simulink library "tpm"  (R2021b)
settings: Solver=VariableStepAuto  StartTime=0.0  StopTime=10.0  RelTol=1e-3
undefined symbols (not defined in the file or in its folder): ENUM_AN_LF, ENUM_AN_LR, ENUM_AN_RF, ENUM_AN_RR, ENUM_POWERSTA_OFF, ENUM_POWERSTA_OFFA, ENUM_POWERSTA_OFFC, ENUM_POWERSTA_ON, ENUM_POWERSTA_READY, ENUM_POWERSTA_STANDBY, ENUM_PWRSTASW_OFF, ENUM_PWRSTASW_OFFA, ENUM_PWRSTASW_OFFCHVCHRG, ENUM_PWRSTASW_STANDBY, FALSE, KTPM_Delay_raw8, KTPM_WhlRotDir_enum_ovrdflg, KTPM_WhlRotDir_enum_ovrdval, TRUE, ZERO_FLOAT, ZERO_INT
libraries: simulink x58, hcu_lib x25, $bdroot x18
(part 8 of 8)

== stateflow chart tpm/TPM/TPMS/TPMS/Learn/AutoLocation/Doublecheck/Chart ==
  (default) -> (junction 18)
  (junction 18) -> (junction 19) [order 1] : [VTPM_SaveToRAM_flg]
  (junction 18) -> (junction 36) [order 2]
  (junction 19) -> (junction 23) : {
      |  VTPM_ChkLFID_raw=VTPM_LFID_raw;
      |  VTPM_ChkRFID_raw=VTPM_RFID_raw;
      |  VTPM_ChkLRID_raw=VTPM_LRID_raw;
      |  VTPM_ChkRRID_raw=VTPM_RRID_raw;
      | }
  (junction 23) -> (junction 36)
  data: VTPM_LFID_raw input; VTPM_RFID_raw input; VTPM_LRID_raw input; VTPM_RRID_raw input; VTPM_ChkLFID_raw output uint32; VTPM_ChkRFID_raw output uint32; VTPM_ChkLRID_raw output uint32; VTPM_ChkRRID_raw output uint32; VTPM_SaveToRAM_flg input

== stateflow chart tpm/TPM/TPMS/TPMS/Learn/AutoLocation/IDIdentify/Subsystem1/Chart1 ==
  state GCal [parallel]
    settings: executionOrder=1
    state NoSignal
      en:G=false;
    state SignalIn
      en:G=true;
    (default) -> NoSignal
    NoSignal -> (junction 17) : [VINP_DATAin_flg]
    (junction 17) -> SignalIn [order 1] : [!Used]
    (junction 17) -> (junction 19) [order 2]
    (junction 19) -> NoSignal [order 2]
    (junction 19) -> SignalIn [order 1] : [VINP_IDin_raw32==IDout]
    SignalIn -> NoSignal
  state IDCheck [parallel]
    settings: executionOrder=2
    state Unused
      en:IDout=0;
      VTPM_S2IDLock_flg=false;
      Used=false;
      IDLock_cnt=0;
    state FlashID
      en:
      IDout=VINP_S2ID_raw;
      Used=true;
      VTPM_S2IDLock_flg=true;
    state VINP_DATAin_flg
      state Used
        en:IDout=VINP_IDin_raw32;
        Used=true;
        IDLock_cnt+=1;
      state Lock
        en:VTPM_S2IDLock_flg=true;
      Used -> Used [order 2] : [VINP_DATAin_flg&&IDout==VINP_IDin_raw32]
      Used -> Lock [order 1] : [IDLock_cnt>=4]
    (default) -> Unused
    Unused -> FlashID [order 1] : [VTPM_FlashIDlock_flg]
    FlashID -> Unused : [VINP_TPMSResButt_flg]
    Unused -> Used [order 2] : [VINP_DATAin_flg]
    Used -> Unused [order 3] : [VTPM_S2timeout_flg==1]
    VINP_DATAin_flg -> Unused : [VINP_TPMSResButt_flg]
  state timecounter [parallel]
    settings: executionOrder=3
    state standby
      en:
      VTPM_S2timeout_flg=0;
      VTPM_timeout_cnt=0;
    state counter
      during:
      VTPM_timeout_cnt=VTPM_timeout_cnt+1;
    state stopcounter
    state timeout
      en:
      VTPM_S2timeout_flg=1;
    (default) -> standby
    (junction 76) -> standby
    (junction 74) -> (junction 76)
    standby -> counter : [Used&&!VTPM_FlashIDlock_flg]
    counter -> standby [order 1] : [!Used||(VINP_DATAin_flg&&IDout==VINP_IDin_raw32)]
    stopcounter -> counter : [VINP_VehSpeed_kph>=20]
    counter -> stopcounter [order 3] : [VINP_VehSpeed_kph<20]
    counter -> timeout [order 2] : [VTPM_timeout_cnt>12000]
    timeout -> (junction 74)
  data: VINP_IDin_raw32 input; VINP_TPMSResButt_flg input; VINP_DATAin_flg input; G output boolean; Used output boolean; VTPM_S2IDLock_flg output boolean; IDout output uint32; VTPM_FlashIDlock_flg input; VINP_S2ID_raw input; VINP_VehSpeed_kph input; IDLock_cnt local uint32; VTPM_timeout_cnt local uint32; VTPM_S2timeout_flg output boolean

== matlab function tpm/TPM/TPMS/TPMS/Learn/AutoLocation/IDIdentify/Subsystem1/Enabled Subsystem1/MATLAB Function ==
  data: C input; S output; Min input; X2 input; X3 input; X4 input; Y2 output; Y3 output; Y4 output; X5 input; X6 input; X7 input; X8 input; X9 input; Y5 output; Y6 output; Y7 output; Y8 output; Y9 output
function [S,Y2,Y3,Y4,Y5,Y6,Y7,Y8,Y9]   = fcn(C,Min,X2,X3,X4,X5,X6,X7,X8,X9)
Y=int16([X2 X3 X4 X5 X6 X7 X8 X9 Min]);
if (C<9)
    S=300;
else
    B=sort(Y);
    D=zeros(1,length(B));
    for i=1:1:length(D)
        if (i~=length(D))
            D(i)=B(i+1)-B(i);
        else
            if (B(length(D))-B(1)>B(1)+96-B(length(D)))
                D(length(D))=B(1)+96-B(length(D));
            else
                D(length(D))=B(length(D))-B(1);
            end
        end
    end

    [K,I]=sort(D);
    S=sum(K(1:7));
end
Y2=Y(2);
Y3=Y(3);
Y4=Y(4);
Y5=Y(5);
Y6=Y(6);
Y7=Y(7);
Y8=Y(8);
Y9=Y(9);

== matlab function tpm/TPM/TPMS/TPMS/Learn/AutoLocation/IDIdentify/Subsystem1/Enabled Subsystem2/MATLAB Function ==
  data: C input; S output; Min input; X2 input; X3 input; X4 input; Y2 output; Y3 output; Y4 output; X5 input; X6 input; X7 input; X8 input; X9 input; Y5 output; Y6 output; Y7 output; Y8 output; Y9 output
function [S,Y2,Y3,Y4,Y5,Y6,Y7,Y8,Y9]   = fcn(C,Min,X2,X3,X4,X5,X6,X7,X8,X9)
Y=int16([X2 X3 X4 X5 X6 X7 X8 X9 Min]);
if (C<9)
    S=300;
else
    B=sort(Y);
    D=zeros(1,length(B));
    for i=1:1:length(D)
        if (i~=length(D))
            D(i)=B(i+1)-B(i);
        else
            if (B(length(D))-B(1)>B(1)+96-B(length(D)))
                D(length(D))=B(1)+96-B(length(D));
            else
                D(length(D))=B(length(D))-B(1);
            end
        end
    end

    [K,I]=sort(D);
    S=sum(K(1:7));
end
Y2=Y(2);
Y3=Y(3);
Y4=Y(4);
Y5=Y(5);
Y6=Y(6);
Y7=Y(7);
Y8=Y(8);
Y9=Y(9);

== matlab function tpm/TPM/TPMS/TPMS/Learn/AutoLocation/IDIdentify/Subsystem1/Enabled Subsystem3/MATLAB Function ==
  data: C input; S output; Min input; X2 input; X3 input; X4 input; Y2 output; Y3 output; Y4 output; X5 input; X6 input; X7 input; X8 input; X9 input; Y5 output; Y6 output; Y7 output; Y8 output; Y9 output
function [S,Y2,Y3,Y4,Y5,Y6,Y7,Y8,Y9]   = fcn(C,Min,X2,X3,X4,X5,X6,X7,X8,X9)
Y=int16([X2 X3 X4 X5 X6 X7 X8 X9 Min]);
if (C<9)
    S=300;
else
    B=sort(Y);
    D=zeros(1,length(B));
    for i=1:1:length(D)
        if (i~=length(D))
            D(i)=B(i+1)-B(i);
        else
            if (B(length(D))-B(1)>B(1)+96-B(length(D)))
                D(length(D))=B(1)+96-B(length(D));
            else
                D(length(D))=B(length(D))-B(1);
            end
        end
    end

    [K,I]=sort(D);
    S=sum(K(1:7));
end
Y2=Y(2);
Y3=Y(3);
Y4=Y(4);
Y5=Y(5);
Y6=Y(6);
Y7=Y(7);
Y8=Y(8);
Y9=Y(9);

== matlab function tpm/TPM/TPMS/TPMS/Learn/AutoLocation/IDIdentify/Subsystem1/Enabled Subsystem5/MATLAB Function ==
  data: C input; S output; Min input; X2 input; X3 input; X4 input; Y2 output; Y3 output; Y4 output; X5 input; X6 input; X7 input; X8 input; X9 input; Y5 output; Y6 output; Y7 output; Y8 output; Y9 output
function [S,Y2,Y3,Y4,Y5,Y6,Y7,Y8,Y9]   = fcn(C,Min,X2,X3,X4,X5,X6,X7,X8,X9)
Y=int16([X2 X3 X4 X5 X6 X7 X8 X9 Min]);
if (C<9)
    S=300;
else
    B=sort(Y);
    D=zeros(1,length(B));
    for i=1:1:length(D)
        if (i~=length(D))
            D(i)=B(i+1)-B(i);
        else
            if (B(length(D))-B(1)>B(1)+96-B(length(D)))
                D(length(D))=B(1)+96-B(length(D));
            else
                D(length(D))=B(length(D))-B(1);
            end
        end
    end

    [K,I]=sort(D);
    S=sum(K(1:7));
end
Y2=Y(2);
Y3=Y(3);
Y4=Y(4);
Y5=Y(5);
Y6=Y(6);
Y7=Y(7);
Y8=Y(8);
Y9=Y(9);

== stateflow chart tpm/TPM/TPMS/TPMS/Send/DATA/Chart ==
  state read
    (default) -> (junction 7) : {
        | VTPM_PreS1Pressure_raw=VINP_FlashLFWheelPress_raw8;
        | VTPM_PreS2Pressure_raw=VINP_FlashRFWheelPress_raw8;
        | VTPM_PreS3Pressure_raw=VINP_FlashLRWheelPress_raw8;
        | VTPM_PreS4Pressure_raw=VINP_FlashRRWheelPress_raw8;
        | VTPM_PreS1Temp_raw=VINP_FlashLFWheelTemp_C;
        | VTPM_PreS2Temp_raw=VINP_FlashRFWheelTemp_C;
        | VTPM_PreS3Temp_raw=VINP_FlashLRWheelTemp_C;
        | VTPM_PreS4Temp_raw=VINP_FlashRRWheelTemp_C;
        | }
    read -> (junction 7) : [VINP_DATAin_flg||VINP_TPMSResButt_flg]
    (junction 7) -> (junction 9) [order 1] : [VINP_IDin_raw32==VTPM_S1ID_raw32&&VTPM_IDLOCK_flg&&VINP_DATAin_flg]
    (junction 7) -> (junction 11) [order 2]
    (junction 9) -> (junction 27) : {VTPM_PreS1Pressure_raw=VINP_Pin_raw8;
        |  VTPM_PreS1Temp_raw=VINP_Tin_raw8;
        |  VTPM_PreS1readdone_flg=true;
        | }
    (junction 11) -> (junction 13) [order 1] : [VINP_IDin_raw32==VTPM_S2ID_raw32&&VTPM_IDLOCK_flg&&VINP_DATAin_flg]
    (junction 11) -> (junction 15) [order 2]
    (junction 13) -> (junction 30) : {VTPM_PreS2Pressure_raw=VINP_Pin_raw8;
        |  VTPM_PreS2Temp_raw=VINP_Tin_raw8;
        |  VTPM_PreS2readdone_flg=true;
        | }
    (junction 15) -> (junction 17) [order 1] : [VINP_IDin_raw32==VTPM_S3ID_raw32&&VTPM_IDLOCK_flg&&VINP_DATAin_flg]
    (junction 15) -> (junction 19) [order 2]
    (junction 17) -> (junction 32) : {VTPM_PreS3Pressure_raw=VINP_Pin_raw8;
        |  VTPM_PreS3Temp_raw=VINP_Tin_raw8;
        |  VTPM_PreS3readdone_flg=true;
        | }
    (junction 19) -> (junction 21) [order 1] : [VINP_IDin_raw32==VTPM_S4ID_raw32&&VTPM_IDLOCK_flg&&VINP_DATAin_flg]
    (junction 19) -> (junction 25) [order 2]
    (junction 21) -> (junction 34) : {VTPM_PreS4Pressure_raw=VINP_Pin_raw8;
        |  VTPM_PreS4Temp_raw=VINP_Tin_raw8;
        |  VTPM_PreS4readdone_flg=true;
        | }
    (junction 34) -> (junction 25)
    (junction 32) -> (junction 34)
    (junction 30) -> (junction 32)
    (junction 27) -> (junction 30)
    (junction 25) -> (junction 82)
    (junction 82) -> (junction 84) [order 1] : [VINP_TPMSResButt_flg]
    (junction 82) -> (junction 88) [order 2]
    (junction 84) -> (junction 86) : {
        | VTPM_PreS1Pressure_raw=0;
        | VTPM_PreS2Pressure_raw=0;
        | VTPM_PreS3Pressure_raw=0;
        | VTPM_PreS4Pressure_raw=0;
        | VTPM_PreS1Temp_raw=215;
        | VTPM_PreS2Temp_raw=215;
        | VTPM_PreS3Temp_raw=215;
        | VTPM_PreS4Temp_raw=215;
        | }
  data: VINP_DATAin_flg input; VTPM_S1ID_raw32 input; VTPM_S2ID_raw32 input; VTPM_S3ID_raw32 input; VTPM_S4ID_raw32 input; VINP_IDin_raw32 input; VTPM_IDLOCK_flg input; VINP_Pin_raw8 input; VTPM_PreS1Pressure_raw output uint8; VTPM_PreS2Pressure_raw output uint8; VTPM_PreS4Pressure_raw output uint8; VTPM_PreS3Pressure_raw output uint8; VINP_Tin_raw8 input; VTPM_PreS1Temp_raw output single; VTPM_PreS2Temp_raw output single; VTPM_PreS3Temp_raw output single; VTPM_PreS4Temp_raw output single; VTPM_PreS1readdone_flg output boolean; VTPM_PreS2readdone_flg output boolean; VTPM_PreS3readdone_flg output boolean; VINP_FlashLFWheelPress_raw8 input; VINP_FlashRFWheelPress_raw8 input; VINP_FlashLRWheelPress_raw8 input; VINP_FlashRRWheelPress_raw8 input; VINP_FlashLFWheelTemp_C input; VINP_FlashRFWheelTemp_C input; VINP_FlashLRWheelTemp_C input; VINP_FlashRRWheelTemp_C input; VINP_TPMSResButt_flg input; VTPM_PreS4readdone_flg output boolean

== matlab function tpm/TPM/TPMS/TPMS/Learn/AutoLocation/IDIdentify/Subsystem3/Enabled Subsystem5/MATLAB Function ==
  data: C input; S output; Min input; X2 input; X3 input; X4 input; Y2 output; Y3 output; Y4 output; X5 input; X6 input; X7 input; X8 input; X9 input; Y5 output; Y6 output; Y7 output; Y8 output; Y9 output
function [S,Y2,Y3,Y4,Y5,Y6,Y7,Y8,Y9]   = fcn(C,Min,X2,X3,X4,X5,X6,X7,X8,X9)
Y=int16([X2 X3 X4 X5 X6 X7 X8 X9 Min]);
if (C<9)
    S=300;
else
    B=sort(Y);
    D=zeros(1,length(B));
    for i=1:1:length(D)
        if (i~=length(D))
            D(i)=B(i+1)-B(i);
        else
            if (B(length(D))-B(1)>B(1)+96-B(length(D)))
                D(length(D))=B(1)+96-B(length(D));
            else
                D(length(D))=B(length(D))-B(1);
            end
        end
    end

    [K,I]=sort(D);
    S=sum(K(1:7));
end
Y2=Y(2);
Y3=Y(3);
Y4=Y(4);
Y5=Y(5);
Y6=Y(6);
Y7=Y(7);
Y8=Y(8);
Y9=Y(9);

== stateflow chart tpm/TPM/TPMS/TPMS/Learn/AutoLocation/IDIdentify/Acceptancerate/Chart2 ==
  state SensorReceived [parallel]
    settings: executionOrder=1
    state VINP_TPMSResButt_flg
      en:
      COUNT1=0;
      ID1_message_ALTU=0;
      C=0;
      STOP=0;
      BackFlg=0;
    state NoSignal
    state VINP_FAT_flg1
      en:
      COUNT1=COUNT1 +1
      C=0
    state VINP_FAT_flg0
      en:
      C=C+1
      ID1_message_ALTU=ID1_message_ALTU+1
    state fivesec
    (default) -> VINP_TPMSResButt_flg
    VINP_TPMSResButt_flg -> NoSignal
    NoSignal -> VINP_TPMSResButt_flg [order 1] : [VINP_TPMSResButt_flg||BackFlg==1]
    NoSignal -> (junction 57) [order 2] : [VINP_DATAin_flg&VINP_IDin_raw32==IDout&S1IDLock&VINP_FAT_flg==1&STOP==0]
    NoSignal -> (junction 61) [order 3] : [VINP_DATAin_flg&VINP_IDin_raw32==IDout&S1IDLock&VINP_FAT_flg==0]
    (junction 57) -> VINP_FAT_flg1
    (junction 61) -> VINP_FAT_flg0
    (junction 97) -> NoSignal : {COUNT1=0,ID1_message_ALTU=0,C=0,STOP=0}
    fivesec -> NoSignal [order 2]
    fivesec -> NoSignal [order 1] : [C==5]{STOP=1;C=0;}
    (junction 105) -> NoSignal : {COUNT1=0,ID1_message_ALTU=0,C=0,STOP=0}
    VINP_FAT_flg1 -> (junction 97) [order 1] : [VINP_TPMSResButt_flg||COUNT1==40||BackFlg==1]
    VINP_FAT_flg0 -> (junction 105) [order 1] : [VINP_TPMSResButt_flg||BackFlg==1]
    VINP_FAT_flg1 -> fivesec [order 2] : [after(500,tick)]
    VINP_FAT_flg0 -> fivesec [order 2] : [after(500,tick)]
  state time_cal [parallel]
    settings: executionOrder=2
    state cal1
      en:
      time_cal=time_cal+1
    state default
      en:
      time_cal=0
      BackFlg=0
    state back
      en:
      BackFlg=1
    (default) -> default
    default -> cal1 : [after(6400,tick)]{BackFlg=0}
    back -> default
    cal1 -> back [order 1] : [VINP_TPMSResButt_flg||time_cal>9]
    cal1 -> cal1 [order 2] : [after(6400,tick)]
  data: VINP_IDin_raw32 input; VINP_TPMSResButt_flg input; VINP_DATAin_flg input; S1IDLock input; COUNT1 output uint8; VINP_FAT_flg input; IDout input; ID1_message_ALTU output uint8; STOP local boolean; C local uint8; time_cal local uint8; BackFlg local boolean

== stateflow chart tpm/TPM/TPMS/TPMS/Learn/AutoLocation/IDIdentify/Acceptancerate/Chart3 ==
  state SensorReceived [parallel]
    settings: executionOrder=1
    state VINP_TPMSResButt_flg
      en:
      COUNT2=0;
      ID2_message_ALTU=0;
      C=0;
      STOP=0;
      BackFlg=0;
    state NoSignal
    state VINP_FAT_flg1
      en:
      COUNT2=COUNT2 +1
      C=0
    state VINP_FAT_flg0
      en:
      C=C+1
      ID2_message_ALTU=ID2_message_ALTU+1
    state fivesec
    (default) -> VINP_TPMSResButt_flg
    VINP_TPMSResButt_flg -> NoSignal
    NoSignal -> VINP_TPMSResButt_flg [order 1] : [VINP_TPMSResButt_flg||BackFlg==1]
    NoSignal -> (junction 57) [order 2] : [VINP_DATAin_flg&VINP_IDin_raw32==IDout&S2IDLock&VINP_FAT_flg==1&STOP==0]
    NoSignal -> (junction 61) [order 3] : [VINP_DATAin_flg&VINP_IDin_raw32==IDout&S2IDLock&VINP_FAT_flg==0]
    (junction 57) -> VINP_FAT_flg1
    (junction 61) -> VINP_FAT_flg0
    (junction 97) -> NoSignal : {COUNT2=0,ID2_message_ALTU=0,C=0,STOP=0}
    fivesec -> NoSignal [order 2]
    fivesec -> NoSignal [order 1] : [C==5]{STOP=1;C=0;}
    (junction 105) -> NoSignal : {COUNT2=0,ID2_message_ALTU=0,C=0,STOP=0}
    VINP_FAT_flg1 -> (junction 97) [order 1] : [VINP_TPMSResButt_flg||COUNT2==40||BackFlg==1]
    VINP_FAT_flg0 -> (junction 105) [order 1] : [VINP_TPMSResButt_flg||BackFlg==1]
    VINP_FAT_flg1 -> fivesec [order 2] : [after(500,tick)]
    VINP_FAT_flg0 -> fivesec [order 2] : [after(500,tick)]
  state time_cal [parallel]
    settings: executionOrder=2
    state cal1
      en:
      time_cal=time_cal+1
    state default
      en:
      time_cal=0
      BackFlg=0
    state back
      en:
      BackFlg=1
    (default) -> default
    default -> cal1 : [after(6400,tick)]{BackFlg=0}
    back -> default
    cal1 -> back [order 1] : [VINP_TPMSResButt_flg||time_cal>9]
    cal1 -> cal1 [order 2] : [after(6400,tick)]
  data: VINP_IDin_raw32 input; VINP_TPMSResButt_flg input; VINP_DATAin_flg input; VINP_FAT_flg input; IDout input; STOP local boolean; C local uint8; ID2_message_ALTU output uint8; COUNT2 output uint8; S2IDLock input; BackFlg local boolean; time_cal local uint8

== stateflow chart tpm/TPM/TPMS/TPMS/Learn/AutoLocation/IDIdentify/IDLOCK ==
  state DataSwitch
    (default) -> (junction 5)
    DataSwitch -> (junction 42)
    (junction 42) -> (junction 5) [order 1] : [VINP_DATAin_flg]
    (junction 5) -> (junction 7) [order 1] : [used1&&VINP_IDin_raw32==IDout1]{DATAout=1;}
    (junction 42) -> (junction 44) [order 2] : {DATAout=0;}
    (junction 5) -> (junction 9) [order 2]
    (junction 9) -> (junction 11) [order 1] : [used2&&VINP_IDin_raw32==IDout2]{DATAout=2;}
    (junction 9) -> (junction 13) [order 2]
    (junction 13) -> (junction 15) [order 1] : [used3&&VINP_IDin_raw32==IDout3]{DATAout=3;}
    (junction 13) -> (junction 17) [order 2]
    (junction 17) -> (junction 19) [order 1] : [used4&&VINP_IDin_raw32==IDout4]{DATAout=4;}
    (junction 17) -> (junction 24) [order 2]
    (junction 24) -> (junction 26) [order 1] : [!used1]{DATAout=1;}
    (junction 24) -> (junction 28) [order 2]
    (junction 28) -> (junction 30) [order 1] : [!used2]{DATAout=2;}
    (junction 28) -> (junction 32) [order 2]
    (junction 32) -> (junction 34) [order 1] : [!used3]{DATAout=3;}
    (junction 32) -> (junction 36) [order 2]
    (junction 36) -> (junction 38) [order 1] : [!used4]{DATAout=4;}
    (junction 36) -> (junction 40) [order 2] : {DATAout=0;}
  data: VINP_DATAin_flg input; used1 input; used2 input; used3 input; used4 input; IDout1 input; IDout2 input; IDout3 input; IDout4 input; VINP_IDin_raw32 input; DATAout output uint8

== stateflow chart tpm/TPM/TPMS/TPMS/Learn/AutoLocation/IDIdentify/Acceptancerate/Chart4 ==
  state SensorReceived [parallel]
    settings: executionOrder=1
    state VINP_TPMSResButt_flg
      en:
      COUNT3=0;
      ID3_message_ALTU=0;
      C=0;
      STOP=0;
      BackFlg=0;
    state NoSignal
    state VINP_FAT_flg1
      en:
      COUNT3=COUNT3 +1
      C=0
    state VINP_FAT_flg0
      en:
      C=C+1
      ID3_message_ALTU=ID3_message_ALTU+1
    state fivesec
    (default) -> VINP_TPMSResButt_flg
    VINP_TPMSResButt_flg -> NoSignal
    NoSignal -> VINP_TPMSResButt_flg [order 1] : [VINP_TPMSResButt_flg||BackFlg==1]
    NoSignal -> (junction 57) [order 2] : [VINP_DATAin_flg&VINP_IDin_raw32==IDout&S3IDLock&VINP_FAT_flg==1&STOP==0]
    NoSignal -> (junction 61) [order 3] : [VINP_DATAin_flg&VINP_IDin_raw32==IDout&S3IDLock&VINP_FAT_flg==0]
    (junction 57) -> VINP_FAT_flg1
    (junction 61) -> VINP_FAT_flg0
    (junction 97) -> NoSignal : {COUNT3=0,ID3_message_ALTU=0,C=0,STOP=0}
    fivesec -> NoSignal [order 2]
    fivesec -> NoSignal [order 1] : [C==5]{STOP=1;C=0;}
    (junction 105) -> NoSignal : {COUNT3=0,ID3_message_ALTU=0,C=0,STOP=0}
    VINP_FAT_flg1 -> (junction 97) [order 1] : [VINP_TPMSResButt_flg||COUNT3==40||BackFlg==1]
    VINP_FAT_flg0 -> (junction 105) [order 1] : [VINP_TPMSResButt_flg||BackFlg==1]
    VINP_FAT_flg1 -> fivesec [order 2] : [after(500,tick)]
    VINP_FAT_flg0 -> fivesec [order 2] : [after(500,tick)]
  state time_cal [parallel]
    settings: executionOrder=2
    state cal1
      en:
      time_cal=time_cal+1
    state default
      en:
      time_cal=0
      BackFlg=0
    state back
      en:
      BackFlg=1
    (default) -> default
    default -> cal1 : [after(6400,tick)]{BackFlg=0}
    back -> default
    cal1 -> back [order 1] : [VINP_TPMSResButt_flg||time_cal>9]
    cal1 -> cal1 [order 2] : [after(6400,tick)]
  data: VINP_IDin_raw32 input; VINP_TPMSResButt_flg input; VINP_DATAin_flg input; S3IDLock input; COUNT3 output uint8; VINP_FAT_flg input; IDout input; ID3_message_ALTU output uint8; STOP local boolean; C local uint8; BackFlg local boolean; time_cal local uint8

== stateflow chart tpm/TPM/TPMS/TPMS/Learn/AutoLocation/IDIdentify/Acceptancerate/Chart5 ==
  state SensorReceived [parallel]
    settings: executionOrder=1
    state VINP_TPMSResButt_flg
      en:
      COUNT4=0;
      ID4_message_ALTU=0;
      C=0;
      STOP=0;
      BackFlg=0;
    state NoSignal
    state VINP_FAT_flg1
      en:
      COUNT4=COUNT4 +1
      C=0
    state VINP_FAT_flg0
      en:
      C=C+1
      ID4_message_ALTU=ID4_message_ALTU+1
    state fivesec
    (default) -> VINP_TPMSResButt_flg
    VINP_TPMSResButt_flg -> NoSignal
    NoSignal -> VINP_TPMSResButt_flg [order 1] : [VINP_TPMSResButt_flg||BackFlg==1]
    NoSignal -> (junction 57) [order 2] : [VINP_DATAin_flg&VINP_IDin_raw32==IDout&S4IDLock&VINP_FAT_flg==1&STOP==0]
    NoSignal -> (junction 61) [order 3] : [VINP_DATAin_flg&VINP_IDin_raw32==IDout&S4IDLock&VINP_FAT_flg==0]
    (junction 57) -> VINP_FAT_flg1
    (junction 61) -> VINP_FAT_flg0
    (junction 97) -> NoSignal : {COUNT4=0,ID4_message_ALTU=0,C=0,STOP=0}
    fivesec -> NoSignal [order 2]
    fivesec -> NoSignal [order 1] : [C==5]{STOP=1;C=0;}
    (junction 105) -> NoSignal : {COUNT4=0,ID4_message_ALTU=0,C=0,STOP=0}
    VINP_FAT_flg1 -> (junction 97) [order 1] : [VINP_TPMSResButt_flg||COUNT4==40||BackFlg==1]
    VINP_FAT_flg0 -> (junction 105) [order 1] : [VINP_TPMSResButt_flg||BackFlg==1]
    VINP_FAT_flg1 -> fivesec [order 2] : [after(500,tick)]
    VINP_FAT_flg0 -> fivesec [order 2] : [after(500,tick)]
  state time_cal [parallel]
    settings: executionOrder=2
    state cal1
      en:
      time_cal=time_cal+1
    state default
      en:
      time_cal=0
      BackFlg=0
    state back
      en:
      BackFlg=1
    (default) -> default
    default -> cal1 : [after(6400,tick)]{BackFlg=0}
    back -> default
    cal1 -> back [order 1] : [VINP_TPMSResButt_flg||time_cal>9]
    cal1 -> cal1 [order 2] : [after(6400,tick)]
  data: VINP_IDin_raw32 input; VINP_TPMSResButt_flg input; VINP_DATAin_flg input; S4IDLock input; COUNT4 output uint8; VINP_FAT_flg input; IDout input; ID4_message_ALTU output uint8; STOP local boolean; C local uint8; BackFlg local boolean; time_cal local uint8

== matlab function tpm/TPM/TPMS/TPMS/Send/DATA/PalarmSwitch ==
  data: LFP output; P1 input; P2 input; P3 input; P4 input; S1L input; S2L input; S3L input; S4L input; RFP output; LRP output; RRP output
function [LFP,RFP,LRP,RRP] = fcn(P1,P2,P3,P4,S1L,S2L,S3L,S4L)
P=[P1 P2 P3 P4];
S=[S1L S2L S3L S4L];
LFP=uint8(0);
RFP=uint8(0);
LRP=uint8(0);
RRP=uint8(0);
for i=1:length(S)
    if S(i)==1
        LFP=uint8(P(i));
    elseif S(i)==2
        RFP=uint8(P(i));
    elseif S(i)==3
        LRP=uint8(P(i));
    elseif S(i)==4
        RRP=uint8(P(i));
    end
end

== matlab function tpm/TPM/TPMS/TPMS/Send/DATA/LPindSwitch ==
  data: LFP output; P1 input; P2 input; P3 input; P4 input; S1L input; S2L input; S3L input; S4L input; RFP output; LRP output; RRP output
function [LFP,RFP,LRP,RRP] = fcn(P1,P2,P3,P4,S1L,S2L,S3L,S4L)
P=[P1 P2 P3 P4];
S=[S1L S2L S3L S4L];
LFP=uint8(0);
RFP=uint8(0);
LRP=uint8(0);
RRP=uint8(0);
for i=1:length(S)
    if S(i)==1
        LFP=uint8(P(i));
    elseif S(i)==2
        RFP=uint8(P(i));
    elseif S(i)==3
        LRP=uint8(P(i));
    elseif S(i)==4
        RRP=uint8(P(i));
    end
end

== stateflow chart tpm/TPM/TPMS/TPMS/Send/DATA/LFSW ==
  state OFF
  state ON
    state Reset_Cail
      en:
      VTPM_LFPindi_enum=0;
      VTPM_LFWheelTemp_C=215;
      VTPM_LFWheelPSW_raw8=93;
    state StandBy
    state Received
      en:VTPM_LFWheelPress_raw8=VINP_Pin_raw8;
      VTPM_LFWheelTemp_C=VTPM_Tin_c;
      VTPM_LFBatWarn_flg=VINP_BatteryLow_flg;
      VTPM_LFP20_raw8=uint8(((double(VTPM_LFWheelPress_raw8)*1.72+151)*(273+20)/(273+double(VTPM_LFWheelTemp_C))-151)/1.72);
      VTPM_LFWheelDebug_flg=true;
      VTPM_LFSensorMode_flg=VINP_FAT_flg;
      VTPM_LFWheelPSW_raw8=VTPM_LFPalarm_raw16;
      VTPM_LFPindi_enum=VTPM_S1LowPindi_enum;
      VTPM_LFSensorFail_flg=false;
      ex:
      VTPM_LFWheelDebug_flg=false;
      VTPM_LFSensorMode_flg=false;
    state PreSenfail
    state SensorFail
      en:VTPM_LFSensorFail_flg=true;
    (default) -> StandBy
    StandBy -> Received [order 1] : [VTPM_LFSW_flg==true]
    StandBy -> Reset_Cail [order 3] : [VINP_TPMSCaliButt_flg||VINP_TPMSResButt_flg]
    Received -> StandBy : [VTPM_LFSW_flg==false]
    Reset_Cail -> StandBy
    PreSenfail -> StandBy [order 2] : [VINP_VehSpeed_kph<25]
    StandBy -> PreSenfail [order 2] : [VINP_VehSpeed_kph>=25&&VTPM_Done_flg]
    PreSenfail -> Received [order 1] : [VTPM_LFSW_flg==true]
    SensorFail -> Received : [VTPM_LFSW_flg==true]
    PreSenfail -> SensorFail [order 3] : [after(48000,tick)]
  (default) -> OFF
  ON -> OFF : [VPMM_PowerSta_enum==ENUM_POWERSTA_OFF||...
      | VPMM_PowerSta_enum==ENUM_POWERSTA_OFFC||...
      | VPMM_PowerSta_enum==ENUM_POWERSTA_OFFA||...
      | VPMM_PowerSta_enum==ENUM_POWERSTA_STANDBY
      | ]
  OFF -> ON : [VPMM_PowerSta_enum==ENUM_POWERSTA_ON||...
      | VPMM_PowerSta_enum==ENUM_POWERSTA_READY]
  data: VTPM_LFSW_flg input; VINP_Pin_raw8 input; VTPM_Tin_c input; VINP_BatteryLow_flg input; VTPM_LFWheelPress_raw8 output uint8; VTPM_LFWheelTemp_C output single; VTPM_LFBatWarn_flg output boolean; VTPM_LFSensorFail_flg output boolean; VPMM_PowerSta_enum input; VTPM_LFP20_raw8 output uint8; VINP_FAT_flg input; VTPM_LFWheelDebug_flg output boolean; VTPM_LFSensorMode_flg output boolean; VTPM_LFWheelPSW_raw8 output uint8; VTPM_LFPalarm_raw16 input; VTPM_LFPindi_enum output uint8; VTPM_S1LowPindi_enum input; ENUM_POWERSTA_ON parameter; ENUM_POWERSTA_READY parameter; VINP_VehSpeed_kph input; VTPM_Done_flg input; ENUM_POWERSTA_OFF parameter; ENUM_POWERSTA_OFFA parameter; ENUM_POWERSTA_OFFC parameter; ENUM_POWERSTA_STANDBY parameter; VINP_TPMSCaliButt_flg input; VINP_TPMSResButt_flg input

== stateflow chart tpm/TPM/TPMS/TPMS/Learn/AutoLocation/WheelPosition/Chart5 ==
  state Start
    state Forward
      en:
      a=(VTPM_RRWpos_raw+Delta);
      b=(VTPM_RRWpos_raw+Delta)/96;
      VTPM_RRWpos_raw=a-b*96;
    state Else
    state Backward
      en:
      a=(VTPM_RRWpos_raw+Delta);
      b=(VTPM_RRWpos_raw+Delta)/96;
      VTPM_RRWpos_raw=a-b*96;
    (default) -> (junction 54) : {VTPM_RRWpos_raw=0; Delta=0; PulseCountBuf=VINP_RRPulseCount_cnt;}
    Start -> (junction 54) : [hasChanged(VINP_RRPulseCount_cnt)]....
        | {Delta=VINP_RRPulseCount_cnt-PulseCountBuf;
        | PulseCountBuf=VINP_RRPulseCount_cnt;}
    (junction 54) -> (junction 47) [order 1] : [VPMM_PowerSta_enum!=ENUM_PWRSTASW_OFF&&....
        |  VPMM_PowerSta_enum!=ENUM_PWRSTASW_OFFCHVCHRG&&...
        |  VPMM_PowerSta_enum!=ENUM_PWRSTASW_OFFA&&....
        |  VPMM_PowerSta_enum!=ENUM_PWRSTASW_STANDBY&&....
        |  VINP_RRPulseCountV_flg==false]
    (junction 47) -> (junction 6) [order 1] : [VTPM_RRWhlRotDir_enum==1]
    (junction 6) -> Forward [order 1] : [Delta>0]
    (junction 54) -> Else [order 2]
    (junction 47) -> (junction 48) [order 2]
    (junction 6) -> (junction 10) [order 2] : [Delta<0]
    (junction 10) -> Forward : {Delta=Delta+256;}
    (junction 48) -> Else [order 2]
    (junction 48) -> (junction 14) [order 1] : [VTPM_RRWhlRotDir_enum==2]
    (junction 14) -> Backward [order 1] : [Delta>0]{Delta=-Delta+96;}
    (junction 14) -> (junction 16) [order 2] : [Delta<0]
    (junction 16) -> Backward : {Delta=-Delta+128;}
  data: VPMM_PowerSta_enum input; VINP_RRPulseCount_cnt input; VINP_RRPulseCountV_flg input; VTPM_RRWhlRotDir_enum input; VTPM_RRWpos_raw output int16; a local int16; b local int16; Delta local int16; PulseCountBuf local int16; ENUM_PWRSTASW_OFF parameter; ENUM_PWRSTASW_OFFA parameter; ENUM_PWRSTASW_OFFCHVCHRG parameter; ENUM_PWRSTASW_STANDBY parameter

== stateflow chart tpm/TPM/TPMS/TPMS/Learn/LowerTirePressureCalibration/WarningPressureLearn5 ==
  state WarningPressureLearn [parallel]
    settings: executionOrder=1
    state Flash
      en:
      VTPM_P2alarm_raw=VINP_FlashRFWheelPSW_raw8;
      SPressindi=VINP_FlashRFPindi_enum;
    state Standby
      en:
      C=0;
      P=0;
      T=0;
      VTPM_P2alarm_raw=93;
      SPressindi=0;
    state Status
      en:
      P=P+VINP_Pin_raw8;
      T=T+VINP_Tin_raw8;
      C=C+1;
    state Calculate
      en:
      Pavg=P>>2;
      Tavg=T>>2;
      Pavg20=(Pavg*1.72+151)*(273+20)/(273+Tavg)-101;
    state Nopass
      en:
      SPressindi=2;
    state Pass
      en:
      SPressindi=1;
      VTPM_P2alarm_raw=(Pavg20*0.8+14-50)/1.72;
    (default) -> (junction 339)
    (junction 339) -> Flash [order 1] : [VTPM_LocationDone_flg]
    (junction 339) -> Standby [order 2]
    Flash -> (junction 329) : [VINP_TPMSResButt_flg||VINP_TPMSCaliButt_flg]
    (junction 329) -> Standby
    Status -> Standby [order 2] : [VINP_TPMSResButt_flg||VINP_TPMSCaliButt_flg||VTPM_S2timeout_flg]
    Status -> Calculate [order 1] : [C>=4]
    Standby -> (junction 217) : [VINP_DATAin_flg&&!VINP_TPMSResButt_flg&&(VTPM_IDLOCK_flg||VTPM_LocationDone_flg)]
    (junction 217) -> Status : [VINP_IDin_raw32==VTPM_S2ID_raw32....
        | &&VINP_Pin_raw8!=0&&VINP_Tin_raw8!=0]
    (junction 235) -> (junction 217)
    Status -> (junction 235) [order 3] : [VINP_DATAin_flg&&C<4]
    Nopass -> Standby : [VINP_TPMSResButt_flg||VINP_TPMSCaliButt_flg]
    Calculate -> (junction 69)
    (junction 69) -> Nopass [order 2]
    (junction 69) -> Pass [order 1] : [Pavg20>245]
    Pass -> Standby : [VINP_TPMSResButt_flg||VINP_TPMSCaliButt_flg]
  data: VINP_Pin_raw8 input; VINP_Tin_raw8 input; VINP_IDin_raw32 input; VINP_DATAin_flg input; VINP_TPMSResButt_flg input; VINP_TPMSCaliButt_flg input; VTPM_IDLOCK_flg input; VTPM_P2alarm_raw output uint8; Pavg20 local uint8; SPressindi output uint8; P local uint16; Pavg local uint8; T local int16; Tavg local int8; VTPM_S2ID_raw32 input; C local uint8; VTPM_LocationDone_flg input; VINP_FlashRFWheelPSW_raw8 input; VINP_FlashRFPindi_enum input; VTPM_S2timeout_flg input

== stateflow chart tpm/TPM/TPMS/TPMS/Learn/AutoLocation/WheelPosition/Chart1 ==
  state Start
    state Forward
      en:
      a=(VTPM_LFWpos_raw+Delta);
      b=(VTPM_LFWpos_raw+Delta)/96;
      VTPM_LFWpos_raw=a-b*96;
    state Else
    state Backward
      en:
      a=(VTPM_LFWpos_raw+Delta);
      b=(VTPM_LFWpos_raw+Delta)/96;
      VTPM_LFWpos_raw=a-b*96;
    (default) -> (junction 54) : {VTPM_LFWpos_raw=0; Delta=0; PulseCountBuf=VINP_LFPulseCount_cnt;}
    Start -> (junction 54) : [hasChanged(VINP_LFPulseCount_cnt)]....
        | {Delta=VINP_LFPulseCount_cnt-PulseCountBuf;
        | PulseCountBuf=VINP_LFPulseCount_cnt;}
    (junction 54) -> (junction 47) [order 1] : [VPMM_PowerSta_enum!=ENUM_PWRSTASW_OFF&&....
        |  VPMM_PowerSta_enum!=ENUM_PWRSTASW_OFFCHVCHRG&&...
        |  VPMM_PowerSta_enum!=ENUM_PWRSTASW_OFFA&&....
        |  VPMM_PowerSta_enum!=ENUM_PWRSTASW_STANDBY&&....
        |  VINP_LFPulseCountV_flg==false]
    (junction 47) -> (junction 6) [order 1] : [VTPM_LFWhlRotDir_enum==1]
    (junction 6) -> Forward [order 1] : [Delta>0]
    (junction 54) -> Else [order 2]
    (junction 47) -> (junction 48) [order 2]
    (junction 6) -> (junction 10) [order 2] : [Delta<0]
    (junction 10) -> Forward : {Delta=Delta+256;}
    (junction 48) -> Else [order 2]
    (junction 48) -> (junction 14) [order 1] : [VTPM_LFWhlRotDir_enum==2]
    (junction 14) -> Backward [order 1] : [Delta>0]{Delta=-Delta+96;}
    (junction 14) -> (junction 16) [order 2] : [Delta<0]
    (junction 16) -> Backward : {Delta=-Delta+128;}
  data: VPMM_PowerSta_enum input; VINP_LFPulseCount_cnt input; VINP_LFPulseCountV_flg input; VTPM_LFWhlRotDir_enum input; VTPM_LFWpos_raw output int16; a local int16; b local int16; Delta local int16; PulseCountBuf local int16; ENUM_PWRSTASW_OFF parameter; ENUM_PWRSTASW_OFFA parameter; ENUM_PWRSTASW_OFFCHVCHRG parameter; ENUM_PWRSTASW_STANDBY parameter

== stateflow chart tpm/TPM/TPMS/TPMS/Learn/LowerTirePressureCalibration/WarningPressureLearn1 ==
  state WarningPressureLearn
    state Flash
      en:
      VTPM_P1alarm_raw=VINP_FlashLFWheelPSW_raw8;
      VTPM_S1pressindi_enum=VINP_FlashLFPindi_enum;
    state Standby
      en:
      C=0;
      P=0;
      T=0;
      VTPM_P1alarm_raw=93;
      VTPM_S1pressindi_enum=0;
    state Status
      en:
      P=P+VINP_Pin_raw8;
      T=T+VINP_Tin_raw8;
      C=C+1;
    state Calculate
      en:
      Pavg=P>>2;
      Tavg=T>>2;
      Pavg20=(Pavg*1.72+151)*(273+20)/(273+Tavg)-101;
    state Nopass
      en:
      VTPM_S1pressindi_enum=2;
    state Pass
      en:
      VTPM_S1pressindi_enum=1;
      VTPM_P1alarm_raw=(Pavg20*0.8+14-50)/1.72;
    (default) -> (junction 328)
    (junction 328) -> Flash [order 1] : [VTPM_LocationDone_flg]
    (junction 328) -> Standby [order 2]
    Flash -> (junction 342) : [VINP_TPMSResButt_flg||VINP_TPMSCaliButt_flg]
    (junction 342) -> Standby
    Status -> Standby [order 2] : [VINP_TPMSResButt_flg||VINP_TPMSCaliButt_flg||VTPM_S1timeout_flg]
    Status -> Calculate [order 1] : [C>=4]
    Standby -> (junction 217) : [VINP_DATAin_flg&&!VINP_TPMSResButt_flg&&(VTPM_IDLOCK_flg||VTPM_LocationDone_flg)]
    (junction 217) -> Status : [VINP_IDin_raw32==VTPM_S1ID_raw32....
        | &&VINP_Pin_raw8!=0&&VINP_Tin_raw8!=0]
    (junction 235) -> (junction 217)
    Status -> (junction 235) [order 3] : [VINP_DATAin_flg&&C<4]
    (junction 69) -> Nopass [order 2]
    Calculate -> (junction 69)
    Nopass -> Standby : [VINP_TPMSResButt_flg||VINP_TPMSCaliButt_flg]
    (junction 69) -> Pass [order 1] : [Pavg20>245]
    Pass -> Standby : [VINP_TPMSResButt_flg||VINP_TPMSCaliButt_flg]
  data: VINP_Pin_raw8 input; VINP_Tin_raw8 input; VINP_IDin_raw32 input; VINP_DATAin_flg input; VINP_TPMSResButt_flg input; VINP_TPMSCaliButt_flg input; VTPM_IDLOCK_flg input; VTPM_P1alarm_raw output uint8; Pavg20 local uint8; VTPM_S1pressindi_enum output uint8; P local uint16; Pavg local uint8; T local int16; Tavg local int8; VTPM_S1ID_raw32 input; C output uint8; VTPM_LocationDone_flg input; VINP_FlashLFWheelPSW_raw8 input; VINP_FlashLFPindi_enum input; VTPM_S1timeout_flg input

== stateflow chart tpm/TPM/TPMS/TPMS/Learn/AutoLocation/IDIdentify/Subsystem7/Chart ==
  state Sample [parallel]
    settings: executionOrder=1
    state DataNotEnough
    state Regisiter
      en:
      C=C+1;
      LFM=LF_PC;
      RFM=RF_PC;
      LRM=LR_PC;
      RRM=RR_PC;
    (default) -> DataNotEnough : {C=0;}
    DataNotEnough -> Regisiter [order 2] : [!VINP_TPMSResButt_flg&&GS]
    Regisiter -> (junction 513) [order 2] : [GS]
    (junction 513) -> (junction 514)
    (junction 514) -> Regisiter
    Regisiter -> DataNotEnough [order 1] : [VINP_TPMSResButt_flg]{C=0;}
    Regisiter -> (junction 528) [order 3] : [VPMM_PowerSta_enum!=ENUM_POWERSTA_ON&&...
        | VPMM_PowerSta_enum!=ENUM_POWERSTA_READY
        | ]
    (junction 528) -> (junction 532) : {C=0;}
    (junction 532) -> DataNotEnough
    DataNotEnough -> DataNotEnough [order 1] : [VINP_TPMSResButt_flg]{C=0;}
  data: VINP_TPMSResButt_flg input; VPMM_PowerSta_enum input; GS input; LR_PC input; LF_PC input; RR_PC input; RF_PC input; LFM output int16; LRM output int16; RRM output int16; RFM output int16; C output uint8; ENUM_POWERSTA_READY parameter; ENUM_POWERSTA_ON parameter

== stateflow chart tpm/TPM/TPMS/TPMS/Send/DATA/LocationSW/Chart1 ==
  state Location [parallel]
    settings: executionOrder=1
    state S1
      en:SLocation=VTPM_S1L_enum;
    state S2
      en:SLocation=VTPM_S2L_enum;
    state S3
      en:SLocation=VTPM_S3L_enum;
    state S4
      en:SLocation=VTPM_S4L_enum;
    state Else
      en:SLocation=0;
    (default) -> (junction 6)
    (junction 6) -> S1 [order 1] : [VTPM_IDLOCK_flg && VINP_DATAin_flg && VINP_IDin_raw32==VTPM_S1ID_raw32]
    Location -> (junction 6)
    (junction 6) -> (junction 7) [order 2]
    (junction 7) -> S2 [order 1] : [VTPM_IDLOCK_flg && VINP_DATAin_flg && VINP_IDin_raw32==VTPM_S2ID_raw32]
    (junction 7) -> (junction 10) [order 2]
    (junction 10) -> S3 [order 1] : [VTPM_IDLOCK_flg && VINP_DATAin_flg && VINP_IDin_raw32==VTPM_S3ID_raw32]
    (junction 10) -> (junction 1) [order 2]
    (junction 1) -> Location.Else [order 2]
    (junction 1) -> S4 [order 1] : [VTPM_IDLOCK_flg && VINP_DATAin_flg && VINP_IDin_raw32==VTPM_S4ID_raw32]
  state Identify [parallel]
    settings: executionOrder=2
    state LF
      en:VTPM_LFSW_flg=true;VTPM_RFSW_flg=false;VTPM_LRSW_flg=false;VTPM_RRSW_flg=false;
    state RF
      en:VTPM_LFSW_flg=false;VTPM_RFSW_flg=true;VTPM_LRSW_flg=false;VTPM_RRSW_flg=false;
    state LR
      en:VTPM_LFSW_flg=false;VTPM_RFSW_flg=false;VTPM_LRSW_flg=true;VTPM_RRSW_flg=false;
    state RR
      en:VTPM_LFSW_flg=false;VTPM_RFSW_flg=false;VTPM_LRSW_flg=false;VTPM_RRSW_flg=true;
    state Else
      en:VTPM_LFSW_flg=false;VTPM_RFSW_flg=false;VTPM_LRSW_flg=false;VTPM_RRSW_flg=false;
    (default) -> (junction 42)
    Identify -> (junction 42)
    (junction 42) -> LF [order 1] : [SLocation==ENUM_AN_LF]
    (junction 42) -> (junction 46) [order 2]
    (junction 46) -> RF [order 1] : [SLocation==ENUM_AN_RF]
    (junction 46) -> (junction 56) [order 2]
    (junction 56) -> LR [order 1] : [SLocation==ENUM_AN_LR]
    (junction 56) -> (junction 47) [order 2]
    (junction 47) -> RR [order 1] : [SLocation==ENUM_AN_RR]
    (junction 47) -> Identify.Else [order 2]
  data: VTPM_S1ID_raw32 input; VTPM_S1L_enum input; VTPM_S2ID_raw32 input; VTPM_S2L_enum input; VTPM_S3ID_raw32 input; VTPM_S3L_enum input; VTPM_S4ID_raw32 input; VTPM_S4L_enum input; VINP_IDin_raw32 input; VINP_DATAin_flg input; VTPM_IDLOCK_flg input; VTPM_LFSW_flg output boolean; VTPM_RFSW_flg output boolean; VTPM_LRSW_flg output boolean; VTPM_RRSW_flg output boolean; SLocation local uint8; ENUM_AN_LF parameter; ENUM_AN_LR parameter; ENUM_AN_RF parameter; ENUM_AN_RR parameter

== matlab function tpm/TPM/TPMS/TPMS/Learn/AutoLocation/Doublecheck/MATLAB Function ==
  data: S1ID input; LFID output; S2ID input; S3ID input; S4ID input; S1L input; S2L input; S3L input; S4L input; VTPM_ALLFin_flg input; RFID output; LRID output; RRID output
function [LFID, RFID, LRID, RRID] = fcn(S1ID, S2ID, S3ID, S4ID, S1L, S2L, S3L, S4L, VTPM_ALLFin_flg)
    LFID = uint32(0);
    RFID = uint32(0);
    LRID = uint32(0);
    RRID = uint32(0);
    
    if VTPM_ALLFin_flg == 1
        ID = [S1ID, S2ID, S3ID, S4ID];
        Location = [S1L, S2L, S3L, S4L];
        
        for i = 1:length(Location)
            if Location(i) == 1
                LFID = uint32(ID(i));
            elseif Location(i) == 2
                RFID = uint32(ID(i));
            elseif Location(i) == 3
                LRID = uint32(ID(i));
            elseif Location(i) == 4
                RRID = uint32(ID(i));
            end
        end
    end
end

== stateflow chart tpm/TPM/TPMS/TPMS/Subsystem/Chart ==
  state WriteChkLFID [parallel]
    settings: executionOrder=1
    (default) -> (junction 131)
    WriteChkLFID -> (junction 131) : [VTPM_SetChkId_flg||VINP_TPMSResButt_flg]
    (junction 131) -> (junction 102) : {
        | VTPM_WriteChkLFID_raw=VTPM_WriteLFID_raw;
        | VTPM_WriteChkRFID_raw=VTPM_WriteRFID_raw;
        | VTPM_WriteChkLRID_raw=VTPM_WriteLRID_raw;
        | VTPM_WriteChkRRID_raw=VTPM_WriteRRID_raw;
        | VTPM_Flashchkdatavalid_flg=1;
        | }
    (junction 102) -> (junction 104) [order 1] : [VINP_TPMSResButt_flg||!VTPM_SetChkId_flg]
    (junction 102) -> (junction 108) [order 2]
    (junction 104) -> (junction 106) : {VTPM_WriteChkLFID_raw=ZERO_INT;
        | VTPM_WriteChkRFID_raw=ZERO_INT;
        | VTPM_WriteChkLRID_raw=ZERO_INT;
        | VTPM_WriteChkRRID_raw=ZERO_INT;
        | VTPM_Flashchkdatavalid_flg=0;
        | }
    (junction 106) -> (junction 108)
  state WriteChkFinLFID [parallel]
    settings: executionOrder=2
    (default) -> (junction 128)
    WriteChkFinLFID -> (junction 128) : [VTPM_CheckFin_flg||VINP_TPMSResButt_flg]
    (junction 128) -> (junction 112) : {VTPM_WriteChkfinLFID_raw=VTPM_WriteLFID_raw;
        | VTPM_WriteChkfinRFID_raw=VTPM_WriteRFID_raw;
        | VTPM_WriteChkfinLRID_raw=VTPM_WriteLRID_raw;
        | VTPM_WriteChkfinRRID_raw=VTPM_WriteRRID_raw;
        | VTPM_Flashdatavalid_flg=1;
        | }
    (junction 112) -> (junction 113) [order 1] : [VINP_TPMSResButt_flg||!VTPM_CheckFin_flg]
    (junction 112) -> (junction 116) [order 2]
    (junction 113) -> (junction 114) : {
        | VTPM_WriteChkfinLFID_raw=ZERO_INT;
        | VTPM_WriteChkfinRFID_raw=ZERO_INT;
        | VTPM_WriteChkfinLRID_raw=ZERO_INT;
        | VTPM_WriteChkfinRRID_raw=ZERO_INT;
        | VTPM_Flashdatavalid_flg=0;
        | }
    (junction 114) -> (junction 116)
  data: VTPM_WriteLFID_raw input; VTPM_WriteRFID_raw input; VTPM_WriteLRID_raw input; VTPM_WriteRRID_raw input; ZERO_INT parameter; VTPM_CheckFin_flg input; VTPM_WriteChkLFID_raw output uint32; VTPM_WriteChkLRID_raw output uint32; VTPM_WriteChkRFID_raw output uint32; VTPM_WriteChkRRID_raw output uint32; VTPM_WriteChkfinLFID_raw output uint32; VTPM_WriteChkfinLRID_raw output uint32; VTPM_WriteChkfinRFID_raw output uint32; VTPM_WriteChkfinRRID_raw output uint32; VINP_TPMSResButt_flg input; VTPM_SetChkId_flg input; VTPM_Flashchkdatavalid_flg output boolean; VTPM_Flashdatavalid_flg output boolean

== matlab function tpm/TPM/TPMS/TPMS/Subsystem/MATLAB Function ==
  data: S1ID input; LFID output; S2ID input; S3ID input; S4ID input; S1L input; S2L input; S3L input; S4L input; set input; RFID output; LRID output; RRID output
function [LFID, RFID, LRID, RRID] = fcn(S1ID, S2ID, S3ID, S4ID, S1L, S2L, S3L, S4L, set)
    LFID = uint32(0);
    RFID = uint32(0);
    LRID = uint32(0);
    RRID = uint32(0);
    
    if set == 1
        ID = [S1ID, S2ID, S3ID, S4ID];
        Location = [S1L, S2L, S3L, S4L];
        
        for i = 1:length(Location)
            if Location(i) == 1
                LFID = uint32(ID(i));
            elseif Location(i) == 2
                RFID = uint32(ID(i));
            elseif Location(i) == 3
                LRID = uint32(ID(i));
            elseif Location(i) == 4
                RRID = uint32(ID(i));
            end
        end
    end
end
